simulink model "assgn_4_model"  (R2021a)
settings: Solver=VariableStepAuto  StartTime=0.0  StopTime=10  RelTol=1e-3
undefined symbols (not defined in the file): A, B, C2, Continuous, K_lqr, Time, x0
libraries: ctrlSharedLib x1
settings Model: Creator=DEVESH  LastModifiedBy=vedan
settings SolverCC: AlgebraicLoopSolver=TrustRegion
settings DebuggingCC: SFMachineParentedDataDiag=warning

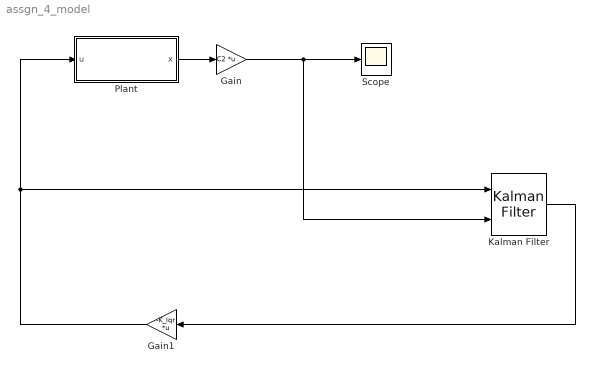
== system assgn_4_model ==
  Gain : Gain  Gain=C2  Multiplication=Matrix(K*u)
  Gain1 : Gain  Gain=-K_lqr  Multiplication=Matrix(K*u)
  Kalman Filter : ctrlSharedLib/Kalman Filter  TimeDomain=Continuous-Time  UseCurrentEstimator=on  ModelSource=Individual A, B, C, D matrices  ModelSourceVariable=ss(0.95,1,1,0,1)  A=A  B=B  C=C2  D=0  NumberOfStates=1  NumberOfInputs=1  NumberOfOutputs=1  InitialEstimateSource=Dialog  X0=x0  P0=10  UseK=off  UseGH=off  NumberOfProcessNoiseInputs=1  G=1  TimeInvariantG=on  H=0  TimeInvariantH=on  Q=diag([0 0 0 0.005])  TimeInvariantQ=on  R=1  TimeInvariantR=on  N=0  TimeInvariantN=on  AddInputPort=on  AddEnablePort=off  OutputEstimatedY=off  OutputP=off  Ts=-1
  Plant : Subsystem
  Scope : Scope
  wires:
  Plant/1(x) -> Gain/1
  Kalman Filter/1 -> Gain1/1
  Gain/1 -> Kalman Filter/2, Scope/1
  Gain1/1 -> Plant/1(u), Kalman Filter/1

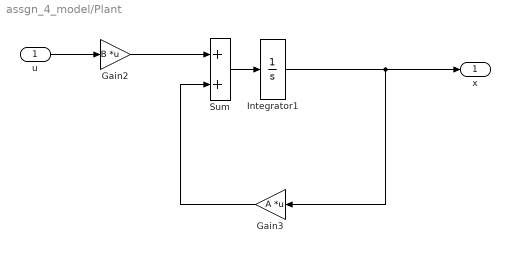
== system assgn_4_model/Plant ==
  u : Inport
  Gain2 : Gain  Gain=B  Multiplication=Matrix(K*u)
  Gain3 : Gain  Gain=A  Multiplication=Matrix(K*u)
  Integrator1 : Integrator  InitialCondition=x0
  Sum : Sum
  x : Outport
  wires:
  Gain2/1 -> Sum/1
  u/1 -> Gain2/1
  Integrator1/1 -> x/1, Gain3/1
  Sum/1 -> Integrator1/1
  Gain3/1 -> Sum/2
